simulink model "AveragingEx"  (R2015a)
settings: Solver=ode45  StartTime=0.0  StopTime=10.0  RelTol=1e-3
libraries: lib_GenTools_Averaging x2, lib_GenTools_WeightedAveraging x1
settings Model: Creator=jlkratz  LastModifiedBy=jlkratz

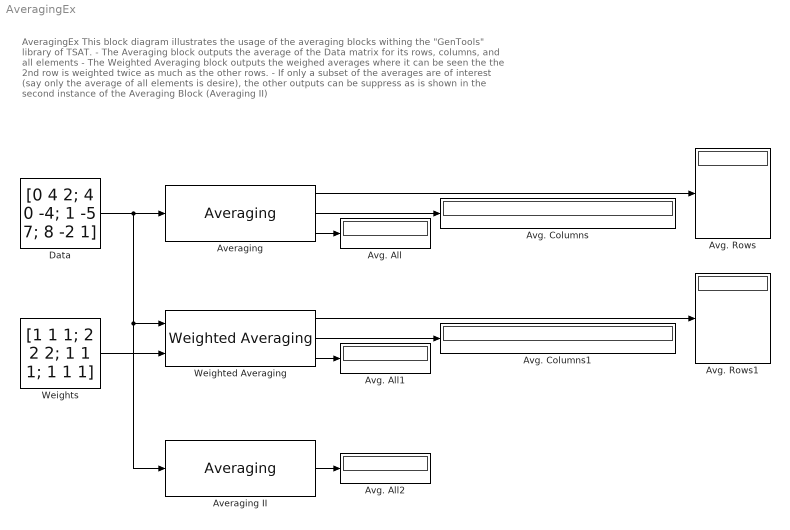
== system AveragingEx ==
  note: AveragingEx
      |
      | This block diagram illustrates the usage of the averaging blocks withing the "GenTools" library of TSAT.
      | - The Averaging block outputs the average of the Data matrix for its rows, columns, and all elements
      | - The Weighted Averaging block outputs the weighed averages where it can be seen the the 2nd row
      | is weighted twice as much as the other rows.
      | - If only a subset of the averages are of interest (say only the average of all elements is desire), the other
      | outputs can be suppress as is shown in the second instance of the Averaging Block (Averaging II)
  Averaging : lib_GenTools_Averaging/Averaging  avg_rows_M=on  avg_cols_M=on  avg_all_M=on  BN_M=gcb
  Averaging II : lib_GenTools_Averaging/Averaging  avg_rows_M=off  avg_cols_M=off  avg_all_M=on  BN_M=gcb
  Avg. All : Display
  Avg. All1 : Display
  Avg. All2 : Display
  Avg. Columns : Display
  Avg. Columns1 : Display
  Avg. Rows : Display
  Avg. Rows1 : Display
  Data : Constant  Value=[0 4 2; 4 0 -4; 1 -5 7; 8 -2 1]
  Weighted Averaging : lib_GenTools_WeightedAveraging/Weighted Averaging  avg_rows_M=on  avg_cols_M=on  avg_all_M=on  BN_M=gcb
  Weights : Constant  Value=[1 1 1; 2 2 2; 1 1 1; 1 1 1]
  wires:
  Data/1 -> Averaging II/1, Weighted Averaging/1, Averaging/1
  Averaging/3 -> Avg. All/1
  Averaging/2 -> Avg. Columns/1
  Averaging/1 -> Avg. Rows/1
  Weights/1 -> Weighted Averaging/2
  Weighted Averaging/2 -> Avg. Columns1/1
  Weighted Averaging/1 -> Avg. Rows1/1
  Weighted Averaging/3 -> Avg. All1/1
  Averaging II/1 -> Avg. All2/1
